simulink model "bh_boat_stabilizer_model"  (R2022b)
settings: Solver=ode15s  StartTime=0.0  StopTime=45  RelTol=1e-6  AbsTol=1e-6  EnableMultiTasking=on
undefined symbols (not defined in the file or in its folder): cage, disk, hull, my_points, sigbuilder_block, stand, X, Y, Z
libraries: sm_lib x37, nesl_utility x18, simulink_extras x18, simulink x1
(part 3 of 3)

== matlab function bh_boat_stabilizer_model/Boat_plant_hand/EOM_SYS/my_A_and_b1 ==
  data: Icage_xx input; A output; Icage_xy input; Icage_xz input; Icage_yy input; Icage_yz input; Icage_zz input; Idisk_xx input; Idisk_xy input; Idisk_xz input; Idisk_yy input; Idisk_yz input; Idisk_zz input; Ihull_zz input; beta input; beta_dot input; g input; m_cage input; m_disk input; m_hull input; phi input; phi_dot input; tau_disk input; tau_hull input; theta input; theta_dot input; y_CG_H_disk input; y_CG_H_hull input; b output
function [A,b] = my_A_and_b(Icage_xx,Icage_xy,Icage_xz,Icage_yy,Icage_yz,Icage_zz,Idisk_xx,Idisk_xy,Idisk_xz,Idisk_yy,Idisk_yz,Idisk_zz,Ihull_zz,beta,beta_dot,g,m_cage,m_disk,m_hull,phi,phi_dot,tau_disk,tau_hull,theta,theta_dot,y_CG_H_disk,y_CG_H_hull)
%#codegen

%    This function was generated by the Symbolic Math Toolbox version 9.2.
%    27-Oct-2022 12:54:24

mt1 = [-Ihull_zz-m_cage.*y_CG_H_disk.^2-m_disk.*y_CG_H_disk.^2-m_hull.*y_CG_H_hull.^2-Icage_zz.*cos(phi).^2-Icage_yz.*sin(phi.*2.0)-Icage_yy.*sin(phi).^2-Idisk_yy.*sin(phi).^2-Idisk_zz.*cos(beta).^2.*cos(phi).^2-Idisk_xx.*cos(phi).^2.*sin(beta).^2-Idisk_yz.*cos(beta).*cos(phi).*sin(phi).*2.0+Idisk_xy.*cos(phi).*sin(beta).*sin(phi).*2.0+Idisk_xz.*cos(beta).*cos(phi).^2.*sin(beta).*2.0,Icage_xz.*cos(phi).*2.0-Idisk_xz.*cos(phi).*2.0+Icage_xy.*sin(phi).*2.0+Idisk_xy.*cos(beta).*sin(phi).*2.0+Idisk_yz.*sin(beta).*sin(phi).*2.0+Idisk_xz.*cos(beta).^2.*cos(phi).*4.0-Idisk_xx.*cos(beta).*cos(phi).*sin(beta).*2.0+Idisk_zz.*cos(beta).*cos(phi).*sin(beta).*2.0,Idisk_yy.*sin(phi).*-2.0-Idisk_yz.*cos(beta).*cos(phi).*2.0+Idisk_xy.*cos(phi).*sin(beta).*2.0];
mt2 = [-Icage_xz.*cos(phi)-Icage_xy.*sin(phi)-Idisk_xy.*cos(beta).*sin(phi)-Idisk_yz.*sin(beta).*sin(phi)-Idisk_xz.*cos(beta).^2.*cos(phi)+Idisk_xz.*cos(phi).*sin(beta).^2+Idisk_xx.*cos(beta).*cos(phi).*sin(beta)-Idisk_zz.*cos(beta).*cos(phi).*sin(beta),Icage_xx.*2.0+Idisk_zz.*2.0+Idisk_xx.*cos(beta).^2.*2.0-Idisk_zz.*cos(beta).^2.*2.0+Idisk_xz.*sin(beta.*2.0).*2.0,Idisk_xy.*cos(beta).*-2.0-Idisk_yz.*sin(beta).*2.0,-Idisk_yy.*sin(phi)-Idisk_yz.*cos(beta).*cos(phi)+Idisk_xy.*cos(phi).*sin(beta),Idisk_xy.*cos(beta).*2.0+Idisk_yz.*sin(beta).*2.0,Idisk_yy.*-2.0];
A = reshape([mt1,mt2],3,3);
if nargout > 1
    et1 = Icage_yz.*theta_dot.^2.*-2.0-Idisk_yz.*beta_dot.^2.*cos(beta).*2.0+Idisk_xy.*beta_dot.^2.*sin(beta).*2.0-Idisk_yz.*theta_dot.^2.*cos(beta).*2.0+Idisk_xy.*theta_dot.^2.*sin(beta).*2.0+Idisk_xz.*beta_dot.*phi_dot.*4.0+Icage_yz.*theta_dot.^2.*cos(phi).^2.*4.0+Icage_yy.*theta_dot.^2.*sin(phi.*2.0)-Icage_zz.*theta_dot.^2.*sin(phi.*2.0)-Idisk_xx.*theta_dot.^2.*sin(phi.*2.0)+Idisk_yy.*theta_dot.^2.*sin(phi.*2.0)-Idisk_xx.*beta_dot.*theta_dot.*cos(phi).*2.0+Idisk_yy.*beta_dot.*theta_dot.*cos(phi).*2.0+Idisk_zz.*beta_dot.*theta_dot.*cos(phi).*2.0+Idisk_yz.*theta_dot.^2.*cos(beta).*cos(phi).^2.*4.0-Idisk_xy.*theta_dot.^2.*cos(phi).^2.*sin(beta).*4.0-Idisk_xz.*beta_dot.*phi_dot.*cos(beta).^2.*8.0+Idisk_xx.*beta_dot.*phi_dot.*sin(beta.*2.0).*2.0-Idisk_zz.*beta_dot.*phi_dot.*sin(beta.*2.0).*2.0-Idisk_yz.*beta_dot.*theta_dot.*cos(beta).*sin(phi).*4.0+Idisk_xy.*beta_dot.*theta_dot.*sin(beta).*sin(phi).*4.0;
    et2 = Idisk_xx.*theta_dot.^2.*cos(beta).^2.*cos(phi).*sin(phi).*2.0-Idisk_zz.*theta_dot.^2.*cos(beta).^2.*cos(phi).*sin(phi).*2.0+Idisk_xx.*beta_dot.*theta_dot.*cos(beta).^2.*cos(phi).*4.0-Idisk_zz.*beta_dot.*theta_dot.*cos(beta).^2.*cos(phi).*4.0+Idisk_xz.*theta_dot.^2.*cos(beta).*cos(phi).*sin(beta).*sin(phi).*4.0+Idisk_xz.*beta_dot.*theta_dot.*cos(beta).*cos(phi).*sin(beta).*8.0;
    et3 = -tau_hull+Icage_xy.*phi_dot.^2.*cos(phi)-Icage_xz.*phi_dot.^2.*sin(phi)-Idisk_xy.*beta_dot.^2.*cos(beta).*cos(phi)+Idisk_xy.*phi_dot.^2.*cos(beta).*cos(phi)-Idisk_yz.*beta_dot.^2.*cos(phi).*sin(beta)+Idisk_yz.*phi_dot.^2.*cos(phi).*sin(beta)+Idisk_yy.*beta_dot.*phi_dot.*cos(phi)+g.*m_cage.*sin(theta).*sqrt(y_CG_H_disk.^2)+g.*m_disk.*sin(theta).*sqrt(y_CG_H_disk.^2)+g.*m_hull.*sin(theta).*sqrt(y_CG_H_hull.^2)-Idisk_xz.*phi_dot.^2.*cos(beta).^2.*sin(phi)+Idisk_xz.*phi_dot.^2.*sin(beta).^2.*sin(phi)+Icage_yz.*phi_dot.*theta_dot.*cos(phi).^2.*2.0+Icage_yy.*phi_dot.*theta_dot.*sin(phi.*2.0)-Icage_zz.*phi_dot.*theta_dot.*sin(phi.*2.0)+Idisk_yy.*phi_dot.*theta_dot.*sin(phi.*2.0)-Icage_yz.*phi_dot.*theta_dot.*sin(phi).^2.*2.0-Idisk_xx.*beta_dot.*phi_dot.*cos(beta).^2.*cos(phi)+Idisk_zz.*beta_dot.*phi_dot.*cos(beta).^2.*cos(phi);
    et4 = Idisk_xx.*beta_dot.*phi_dot.*cos(phi).*sin(beta).^2-Idisk_zz.*beta_dot.*phi_dot.*cos(phi).*sin(beta).^2+Idisk_yz.*phi_dot.*theta_dot.*cos(beta).*cos(phi).^2.*2.0-Idisk_xy.*phi_dot.*theta_dot.*cos(phi).^2.*sin(beta).*2.0-Idisk_yz.*phi_dot.*theta_dot.*cos(beta).*sin(phi).^2.*2.0+Idisk_xy.*phi_dot.*theta_dot.*sin(beta).*sin(phi).^2.*2.0-Idisk_xz.*beta_dot.*theta_dot.*cos(beta).^2.*cos(phi).^2.*2.0+Idisk_xz.*beta_dot.*theta_dot.*cos(phi).^2.*sin(beta).^2.*2.0+Idisk_xx.*phi_dot.^2.*cos(beta).*sin(beta).*sin(phi)-Idisk_zz.*phi_dot.^2.*cos(beta).*sin(beta).*sin(phi)-Idisk_yz.*beta_dot.*theta_dot.*cos(phi).*sin(beta).*sin(phi).*2.0+Idisk_xx.*beta_dot.*theta_dot.*cos(beta).*cos(phi).^2.*sin(beta).*2.0-Idisk_zz.*beta_dot.*theta_dot.*cos(beta).*cos(phi).^2.*sin(beta).*2.0-Idisk_zz.*phi_dot.*theta_dot.*cos(beta).^2.*cos(phi).*sin(phi).*2.0-Idisk_xx.*phi_dot.*theta_dot.*cos(phi).*sin(beta).^2.*sin(phi).*2.0-Idisk_xz.*beta_dot.*phi_dot.*cos(beta).*cos(phi).*sin(beta).*4.0;
    et5 = Idisk_xy.*beta_dot.*theta_dot.*cos(beta).*cos(phi).*sin(phi).*-2.0+Idisk_xz.*phi_dot.*theta_dot.*cos(beta).*cos(phi).*sin(beta).*sin(phi).*4.0;
    mt3 = [et3+et4+et5;et1+et2];
    mt4 = [tau_disk.*-2.0+Idisk_xz.*phi_dot.^2.*2.0-Idisk_xz.*phi_dot.^2.*cos(beta).^2.*4.0+Idisk_xx.*phi_dot.^2.*sin(beta.*2.0)-Idisk_zz.*phi_dot.^2.*sin(beta.*2.0)-Idisk_xz.*theta_dot.^2.*cos(phi).^2.*2.0-Idisk_xx.*phi_dot.*theta_dot.*cos(phi).*2.0+Idisk_yy.*phi_dot.*theta_dot.*cos(phi).*2.0+Idisk_zz.*phi_dot.*theta_dot.*cos(phi).*2.0+Idisk_xz.*theta_dot.^2.*cos(beta).^2.*cos(phi).^2.*4.0+Idisk_yz.*theta_dot.^2.*cos(phi).*sin(beta).*sin(phi).*2.0-Idisk_yz.*phi_dot.*theta_dot.*cos(beta).*sin(phi).*4.0+Idisk_xy.*phi_dot.*theta_dot.*sin(beta).*sin(phi).*4.0-Idisk_xx.*theta_dot.^2.*cos(beta).*cos(phi).^2.*sin(beta).*2.0+Idisk_zz.*theta_dot.^2.*cos(beta).*cos(phi).^2.*sin(beta).*2.0+Idisk_xx.*phi_dot.*theta_dot.*cos(beta).^2.*cos(phi).*4.0-Idisk_zz.*phi_dot.*theta_dot.*cos(beta).^2.*cos(phi).*4.0+Idisk_xy.*theta_dot.^2.*cos(beta).*cos(phi).*sin(phi).*2.0+Idisk_xz.*phi_dot.*theta_dot.*cos(beta).*cos(phi).*sin(beta).*8.0];
    b = [mt3;mt4];
end
